simulink model "feedback_harness_pidzg"  (R2013a)
settings: Solver=ode45  StartTime=0.0  StopTime=10  RelTol=1e-3
settings Model: ModifiedByFormat=The MathWorks Inc.  Creator=The MathWorks Inc.  LastModifiedBy=The MathWorks Inc.
settings DataIOCC: SaveOutput=off  SaveTime=off
settings OptimizationCC: ExpressionDepthLimit=2147483647  LifeSpan=1
settings DebuggingCC: FcnCallInpInsideContextMsg=EnableAllAsWarning
settings GRTTargetCC: CombineOutputUpdateFcns=off  GRTInterface=on

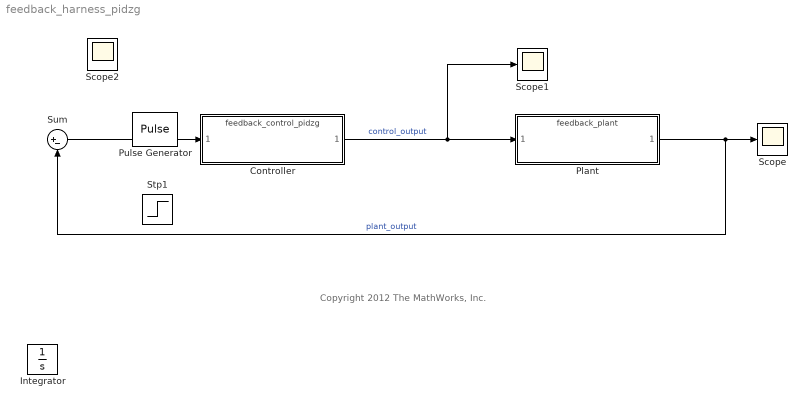
== system feedback_harness_pidzg ==
  note: Copyright 2012 The MathWorks, Inc.
  Controller : ModelReference  ModelNameDialog=feedback_control_pidzg.slx  SimulationMode=Normal  ModelReferenceVersion=1.47  CopyOfModelName=feedback_control_pidzg.slx  DefaultDataLogging=on
  Integrator : Integrator
  Plant : ModelReference  ModelNameDialog=feedback_plant  SimulationMode=Normal  ModelReferenceVersion=1.22  CopyOfModelName=feedback_plant  DefaultDataLogging=on
  Scope : Scope
      settings: YMin=0  YMax=1.4
  Scope1 : Scope
      settings: YMin=0  YMax=1.4
  Scope2 : Scope
      settings: YMin=0  YMax=1.4  SaveName=ScopeData2
  Sum : Sum  Inputs=|+-
  Pulse Generator : DiscretePulseGenerator  IOType=siggen  PulseType=Time based  Period=4  PulseWidth=50
  Stp1 : Step  IOType=siggen  Time=4  SampleTime=0
  wires:
  Controller/1 -> Scope1/1, Plant/1  "control_output"
  Plant/1 -> Scope/1, Sum/2  "plant_output"
  Sum/1 -> Controller/1
